simulink model "PIDControlledSimulinkModel"  (R2024b)
settings: Solver=ode5  StartTime=0.0  StopTime=10000.0  FixedStep=0.1  RelTol=1e-3
values from neighbouring files (symbols this model uses):
  K = 300    [PID_var.m]
  Kp = (1.2*T)/(K*L)    (= 0.012)    [PID_var.m]
  L = 500    [PID_var.m]
  T = 1500    [PID_var.m]
  Td = L/2    (= 250)    [PID_var.m]
  Ti = T*L    (= 750000)    [PID_var.m]
settings Model: Creator=EthanK  LastModifiedBy=EthanK

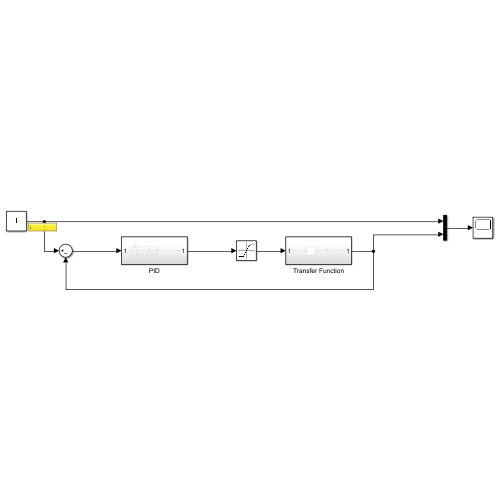
[thumbnail: Simulink's stored preview of the top-level diagram]
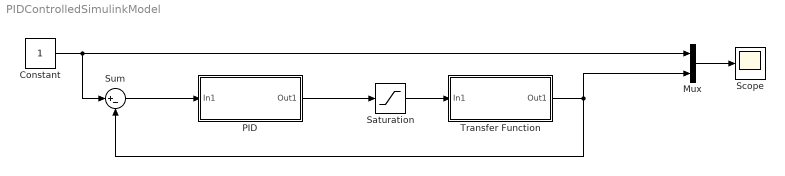
== system PIDControlledSimulinkModel ==
  Constant : Constant
  Mux : Mux  Inputs=2
  PID : Subsystem
  Saturation : Saturate  UpperLimit=1  LowerLimit=0
  Scope : Scope
  Sum : Sum  Inputs=|+-
  Transfer Function : Subsystem
  wires:
  Mux/1 -> Scope/1
  Transfer Function/1(Out1) -> Sum/2, Mux/2
  Constant/1 -> Sum/1, Mux/1
  Saturation/1 -> Transfer Function/1(In1)
  Sum/1 -> PID/1(In1)
  PID/1(Out1) -> Saturation/1

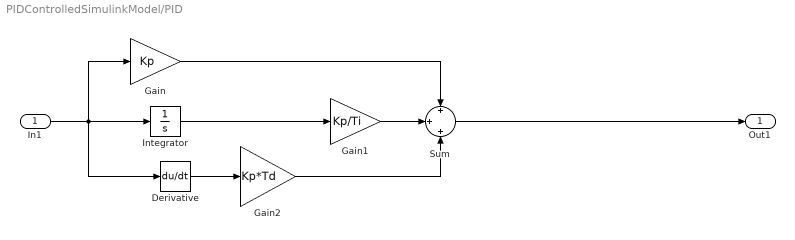
== system PIDControlledSimulinkModel/PID ==
  In1 : Inport
  Derivative : Derivative
  Gain : Gain  Gain=Kp
  Gain1 : Gain  Gain=Kp/Ti
  Gain2 : Gain  Gain=Kp*Td
  Integrator : Integrator
  Sum : Sum  Inputs=+|+|+
  Out1 : Outport
  wires:
  In1/1 -> Derivative/1, Integrator/1, Gain/1
  Sum/1 -> Out1/1
  Gain1/1 -> Sum/2
  Gain/1 -> Sum/1
  Integrator/1 -> Gain1/1
  Gain2/1 -> Sum/3
  Derivative/1 -> Gain2/1

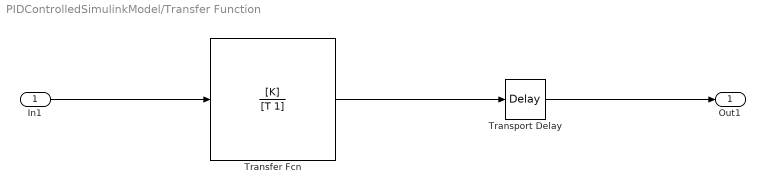
== system PIDControlledSimulinkModel/Transfer Function ==
  In1 : Inport
  Transfer Fcn : TransferFcn  Numerator=[K]  Denominator=[T 1]
  Transport Delay : TransportDelay  DelayTime=L
  Out1 : Outport
  wires:
  In1/1 -> Transfer Fcn/1
  Transport Delay/1 -> Out1/1
  Transfer Fcn/1 -> Transport Delay/1
